simulink model "PID_Control_model"  (R2023a)
settings: Solver=VariableStepAuto  StartTime=0.0  StopTime=2  RelTol=1e-3
values from neighbouring files (symbols this model uses):
  amp = 0.01    [MS_PID_Control.m]    (also in PID_Control.m)
settings Model: Creator=z'k'x  LastModifiedBy=z'k'x

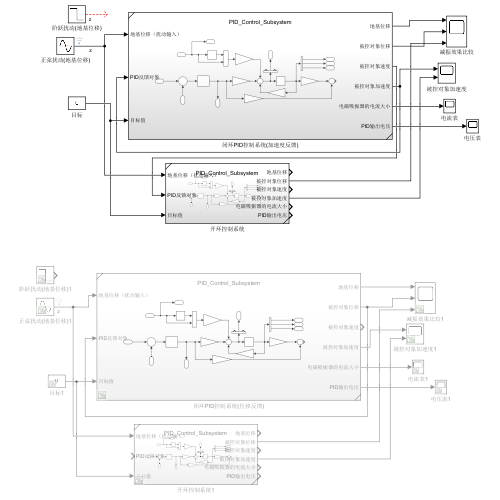
[thumbnail: Simulink's stored preview of the top-level diagram]
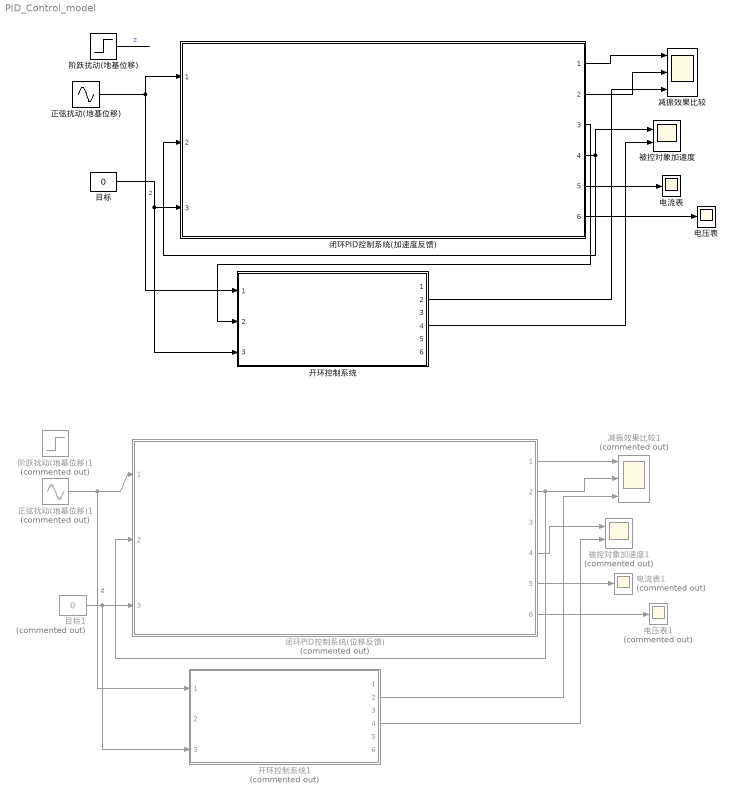
== system PID_Control_model ==
  减振效果比较 : Scope  NumInputPorts=3
  减振效果比较1 : Scope  Commented=on  NumInputPorts=3
  开环控制系统 : Subsystem  VariantControl=Choice  ReferencedSubsystem=PID_Control_Subsystem
  开环控制系统1 : Subsystem  Commented=on  VariantControl=Choice  ReferencedSubsystem=PID_Control_Subsystem
  正弦扰动(地基位移) : Sin  Amplitude=amp  Frequency=17.38*pi  SampleTime=0
  正弦扰动(地基位移)1 : Sin  Commented=on  Amplitude=amp  Frequency=17.38*pi  SampleTime=0
  电压表 : Scope
  电压表1 : Scope  Commented=on
  电流表 : Scope
  电流表1 : Scope  Commented=on
  目标 : Constant  Value=0
  目标1 : Constant  Commented=on  Value=0
  被控对象加速度 : Scope  NumInputPorts=2
  被控对象加速度1 : Scope  Commented=on  NumInputPorts=2
  闭环PID控制系统(位移反馈) : Subsystem  Commented=on  VariantControl=Choice  ReferencedSubsystem=PID_Control_Subsystem
  闭环PID控制系统(加速度反馈) : Subsystem  VariantControl=Choice  ReferencedSubsystem=PID_Control_Subsystem
  阶跃扰动(地基位移) : Step  Time=0.1  Before=0.01  After=0  SampleTime=0
  阶跃扰动(地基位移)1 : Step  Commented=on  Time=0.1  Before=0.01  After=0  SampleTime=0
  wires:
  正弦扰动(地基位移)/1 -> 开环控制系统/1, 闭环PID控制系统(加速度反馈)/1  "z"
  闭环PID控制系统(加速度反馈)/5 -> 电流表/1
  闭环PID控制系统(加速度反馈)/6 -> 电压表/1
  闭环PID控制系统(加速度反馈)/4 -> 被控对象加速度/1, 闭环PID控制系统(加速度反馈)/2
  闭环PID控制系统(加速度反馈)/1 -> 减振效果比较/1
  闭环PID控制系统(加速度反馈)/2 -> 减振效果比较/2
  开环控制系统/2 -> 减振效果比较/3
  开环控制系统/4 -> 被控对象加速度/2
  开环控制系统1/4 -> 被控对象加速度1/2
  开环控制系统1/2 -> 减振效果比较1/3
  闭环PID控制系统(位移反馈)/2 -> 闭环PID控制系统(位移反馈)/2, 减振效果比较1/2
  闭环PID控制系统(位移反馈)/1 -> 减振效果比较1/1
  闭环PID控制系统(位移反馈)/6 -> 电压表1/1
  闭环PID控制系统(位移反馈)/5 -> 电流表1/1
  正弦扰动(地基位移)1/1 -> 开环控制系统1/1, 闭环PID控制系统(位移反馈)/1  "z"
  闭环PID控制系统(加速度反馈)/3 -> 开环控制系统/2
  闭环PID控制系统(位移反馈)/4 -> 被控对象加速度1/1
  目标1/1 -> 开环控制系统1/3, 闭环PID控制系统(位移反馈)/3
  阶跃扰动(地基位移)/1 -> ?  "z"
  目标/1 -> 开环控制系统/3, 闭环PID控制系统(加速度反馈)/3
